simulink model "exp3_5_STATE_SPACE_LQR"  (R2020b)
settings: Solver=FixedStepDiscrete  StartTime=0.0  StopTime=10  FixedStep=Ts  RelTol=1e-3
undefined symbols (not defined in the file): denH_w, DiscIntNeverNeededParam, enable_integral_action, K_ih, K_ss, National_Instruments, Nu, numH_w, Nx, PCI, sens, step_height, step_start_time, Ts
libraries: sldrtlib x4, simulink x3
settings Model: ExtModeTrigDuration=100000  Creator=umbe  LastModifiedBy=irong
settings RTWCC: Description=Simulink Desktop Real-Time  SystemTargetFile=sldrt.tlc  TemplateMakefile=sldrt.tmf  RTWCompilerOptimization=on
settings CodeAppCC: MaxIdLength=95
settings SimulinkDesktopRealTimeCC: TargetPreCompLibLocation=D:\MATLAB\R2020b\toolbox\sldrt\lib\win64

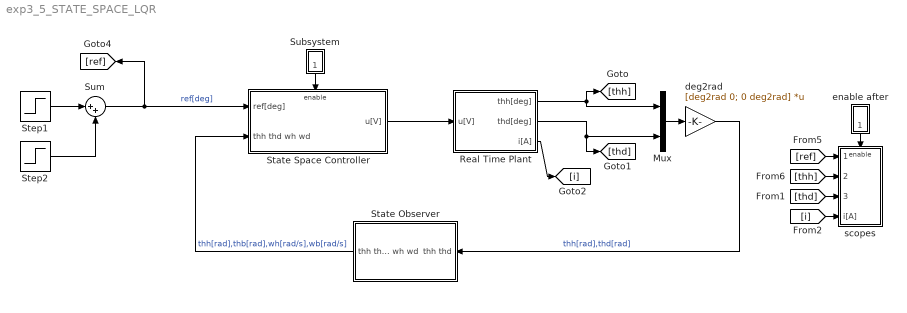
== system exp3_5_STATE_SPACE_LQR ==
  Mux : Mux  Inputs=2
  Real Time Plant : Subsystem
  State Observer : Subsystem
  State Space Controller : Subsystem
  Step1 : Step  Time=step_start_time  After=step_height  SampleTime=0
  Step2 : Step  Time=step_start_time+5  After=-step_height  SampleTime=0
  Subsystem : Subsystem
  Sum : Sum  Inputs=|++
  deg2rad : Gain  Gain=[deg2rad 0; 0 deg2rad]  Multiplication=Matrix(K*u) (u vector)
  enable after : Subsystem
  scopes : Subsystem
  wires:
  [ref] -> scopes/1(ref[deg])
  [thh] -> scopes/2(thh[deg])
  [thd] -> scopes/3(thd[deg])
  [i] -> scopes/4(i[A])
  enable after/1(1.0 s) -> scopes/Enable
  Real Time Plant/1(thh[deg]) -> Mux/1, [thh]
  Real Time Plant/2(thd[deg]) -> Mux/2, [thd]
  Subsystem/1(0.8) -> State Space Controller/Enable
  deg2rad/1 -> State Observer/1(thh thd)  "thh[rad],thd[rad]"
  Mux/1 -> deg2rad/1
  State Space Controller/1(u[V]) -> Real Time Plant/1(u[V])
  State Observer/1(thh thd wh wd) -> State Space Controller/2(thh thd wh wd)  "thh[rad],thb[rad],wh[rad/s],wb[rad/s]"
  Sum/1 -> State Space Controller/1(ref[deg]), [ref]  "ref[deg]"
  Real Time Plant/3(i[A]) -> [i]
  Step2/1 -> Sum/2
  Step1/1 -> Sum/1

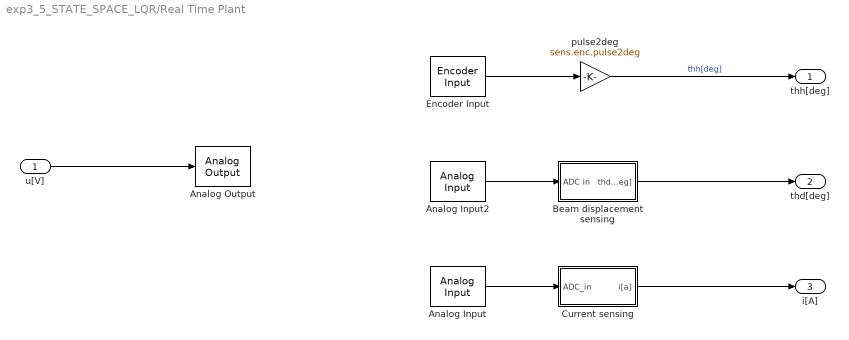
== system exp3_5_STATE_SPACE_LQR/Real Time Plant ==
  u[V] : Inport
  Analog Input : sldrtlib/Analog Input  SampleTime=Ts  MaxMissedTicks=10  ShowMissedTicks=off  YieldWhenWaiting=off  DrvName=National_Instruments/PCI-6221  DrvAddress=4294967295  DrvOptions=[0 0 0 2 0]  Channels=[1 2]  RangeMode=1  VoltRange=1  DataType=1
      settings: AttributesFormatString=National Instruments\nPCI-6221 [auto]
  Analog Input2 : sldrtlib/Analog Input  SampleTime=Ts  MaxMissedTicks=10  ShowMissedTicks=off  YieldWhenWaiting=off  DrvName=National_Instruments/PCI-6221  DrvAddress=4294967295  DrvOptions=[0 0 0 2 0]  Channels=[3,4]  RangeMode=1  VoltRange=2  DataType=1
      settings: AttributesFormatString=National Instruments\nPCI-6221 [auto]
  Analog Output : sldrtlib/Analog Output  SampleTime=Ts  MaxMissedTicks=10  ShowMissedTicks=off  YieldWhenWaiting=off  DrvName=National_Instruments/PCI-6221  DrvAddress=4294967295  DrvOptions=[0 0 0 2 0]  Channels=1  RangeMode=1  VoltRange=1  InitialValue=0  FinalValue=0
      settings: AttributesFormatString=National Instruments\nPCI-6221 [auto]
  Beam displacement sensing : Subsystem
  Current sensing : Subsystem
  Encoder Input : sldrtlib/Encoder Input  SampleTime=Ts  MaxMissedTicks=10  ShowMissedTicks=off  YieldWhenWaiting=off  DrvName=National_Instruments/PCI-6221  DrvAddress=4294967295  DrvOptions=[0 0 0 2 0]  Channels=1  QuadMode=3  IndexPulse=1  InputFilter=Inf  DataType=1
      settings: AttributesFormatString=National Instruments\nPCI-6221 [auto]
  pulse2deg : Gain  Gain=sens.enc.pulse2deg
  thh[deg] : Outport
  thd[deg] : Outport  Port=2
  i[A] : Outport  Port=3
  wires:
  pulse2deg/1 -> thh[deg]/1  "thh[deg]"
  Beam displacement sensing/1(thd[deg]) -> thd[deg]/1
  Analog Input/1 -> Current sensing/1(ADC_in)
  Analog Input2/1 -> Beam displacement sensing/1(ADC in)
  u[V]/1 -> Analog Output/1
  Encoder Input/1 -> pulse2deg/1
  Current sensing/1(i[a]) -> i[A]/1

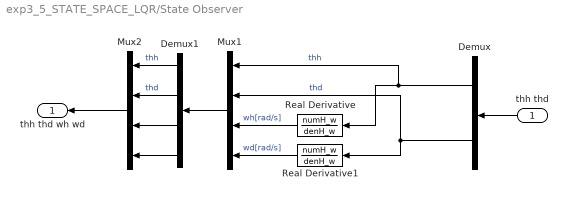
== system exp3_5_STATE_SPACE_LQR/State Observer ==
  thh thd : Inport
  Demux : Demux  Outputs=2
  Demux1 : Demux
  Mux1 : Mux
  Mux2 : Mux
  Real Derivative : TransferFcn  Numerator=numH_w  Denominator=denH_w
  Real Derivative1 : TransferFcn  Numerator=numH_w  Denominator=denH_w
  thh thd wh wd : Outport
  wires:
  Demux1/4 -> Mux2/4
  Demux1/3 -> Mux2/3
  Demux1/2 -> Mux2/2  "thd"
  Demux1/1 -> Mux2/1  "thh"
  Mux1/1 -> Demux1/1
  Mux2/1 -> thh thd wh wd/1
  Demux/2 -> Real Derivative1/1, Mux1/2  "thd"
  Real Derivative1/1 -> Mux1/4  "wd[rad/s]"
  thh thd/1 -> Demux/1
  Demux/1 -> Mux1/1, Real Derivative/1  "thh"
  Real Derivative/1 -> Mux1/3  "wh[rad/s]"

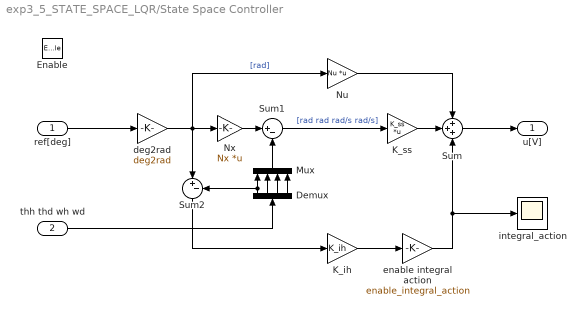
== system exp3_5_STATE_SPACE_LQR/State Space Controller ==
  ref[deg] : Inport
  thh thd wh wd : Inport  Port=2
  Enable : EnablePort
  Demux : Demux
  K_ih : Gain  Gain=K_ih
  K_ss : Gain  Gain=K_ss  Multiplication=Matrix(K*u) (u vector)
  Mux : Mux
  Nu : Gain  Gain=Nu  Multiplication=Matrix(K*u) (u vector)
  Nx : Gain  Gain=Nx  Multiplication=Matrix(K*u) (u vector)
  Sum : Sum  Inputs=+++
  Sum1 : Sum  Inputs=|+-
  Sum2 : Sum  Inputs=|+-
  deg2rad : Gain  Gain=deg2rad
  enable integral action : Gain  Gain=enable_integral_action
  integral_action : Scope
  u[V] : Outport
  wires:
  enable integral action/1 -> integral_action/1, Sum/3
  K_ih/1 -> enable integral action/1
  Sum2/1 -> K_ih/1
  Mux/1 -> Sum1/2
  thh thd wh wd/1 -> Demux/1
  Demux/4 -> Mux/4
  Demux/3 -> Mux/3
  Demux/2 -> Mux/2
  Demux/1 -> Sum2/2, Mux/1
  Sum1/1 -> K_ss/1  "[rad rad rad/s rad/s]"
  Sum/1 -> u[V]/1
  Nu/1 -> Sum/1
  ref[deg]/1 -> deg2rad/1
  Nx/1 -> Sum1/1
  K_ss/1 -> Sum/2
  deg2rad/1 -> Sum2/1, Nu/1, Nx/1  "[rad]"

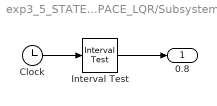
== system exp3_5_STATE_SPACE_LQR/Subsystem ==
  Clock : Clock
  Interval Test : simulink/Logic and Bit Operations/Interval Test  IntervalClosedRight=on  uplimit=inf  IntervalClosedLeft=on  lowlimit=0.8  OutDataTypeStr=boolean
  0.8 : Outport
  wires:
  Interval Test/1 -> 0.8/1
  Clock/1 -> Interval Test/1

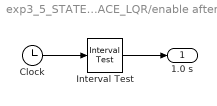
== system exp3_5_STATE_SPACE_LQR/enable after ==
  Clock : Clock
  Interval Test : simulink/Logic and Bit Operations/Interval Test  IntervalClosedRight=on  uplimit=inf  IntervalClosedLeft=on  lowlimit=1  OutDataTypeStr=boolean
  1.0 s : Outport
  wires:
  Clock/1 -> Interval Test/1
  Interval Test/1 -> 1.0 s/1

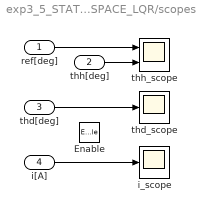
== system exp3_5_STATE_SPACE_LQR/scopes ==
  ref[deg] : Inport
  thh[deg] : Inport  Port=2
  thd[deg] : Inport  Port=3
  i[A] : Inport  Port=4
  Enable : EnablePort
  i_scope : Scope
  thd_scope : Scope
  thh_scope : Scope  NumInputPorts=2
  wires:
  ref[deg]/1 -> thh_scope/1
  thh[deg]/1 -> thh_scope/2
  i[A]/1 -> i_scope/1
  thd[deg]/1 -> thd_scope/1

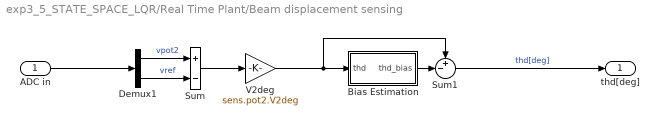
== system exp3_5_STATE_SPACE_LQR/Real Time Plant/Beam displacement sensing ==
  ADC in : Inport
  Bias Estimation : Subsystem
  Demux1 : Demux  Outputs=2
  Sum : Sum  Inputs=+-
  Sum1 : Sum  Inputs=+-|
  V2deg : Gain  Gain=sens.pot2.V2deg
  thd[deg] : Outport
  wires:
  ADC in/1 -> Demux1/1
  V2deg/1 -> Bias Estimation/1(thd), Sum1/1
  Sum1/1 -> thd[deg]/1  "thd[deg]"
  Demux1/2 -> Sum/2  "vref"
  Demux1/1 -> Sum/1  "vpot2"
  Sum/1 -> V2deg/1
  Bias Estimation/1(thd_bias) -> Sum1/2

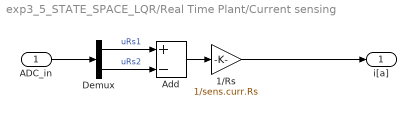
== system exp3_5_STATE_SPACE_LQR/Real Time Plant/Current sensing ==
  ADC_in : Inport
  1/Rs : Gain  Gain=1/sens.curr.Rs
  Add : Sum  Inputs=+-
  Demux : Demux  Outputs=2
  i[a] : Outport
  wires:
  Demux/1 -> Add/1  "uRs1"
  Demux/2 -> Add/2  "uRs2"
  Add/1 -> 1/Rs/1
  ADC_in/1 -> Demux/1
  1/Rs/1 -> i[a]/1

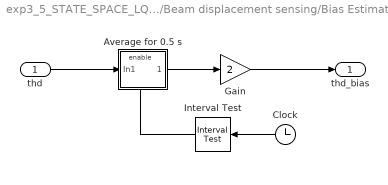
== system exp3_5_STATE_SPACE_LQR/Real Time Plant/Beam displacement sensing/Bias Estimation ==
  thd : Inport
  Average for 0.5 s : Subsystem
  Clock : Clock
  Gain : Gain  Gain=2
  Interval Test : simulink/Logic and Bit Operations/Interval Test  IntervalClosedRight=on  uplimit=0.7  IntervalClosedLeft=on  lowlimit=0.2  OutDataTypeStr=boolean
  thd_bias : Outport
  wires:
  Gain/1 -> thd_bias/1
  Average for 0.5 s/1(Out1) -> Gain/1
  Clock/1 -> Interval Test/1
  thd/1 -> Average for 0.5 s/1(In1)
  Interval Test/1 -> Average for 0.5 s/Enable

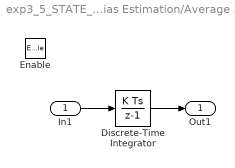
== system exp3_5_STATE_SPACE_LQR/Real Time Plant/Beam displacement sensing/Bias Estimation/Average for 0.5 s ==
  In1 : Inport
  Enable : EnablePort
  Discrete-Time Integrator : DiscreteIntegrator  SampleTime=Ts  ICPrevOutput=DiscIntNeverNeededParam  ICPrevScaledInput=DiscIntNeverNeededParam
  Out1 : Outport
  wires:
  Discrete-Time Integrator/1 -> Out1/1
  In1/1 -> Discrete-Time Integrator/1
